simulink model "Series_RLC"  (R2020b)
settings: Solver=VariableStepAuto  StartTime=0.0  StopTime=0.1  RelTol=1e-3
settings Model: Creator=anubh  LastModifiedBy=anubh
settings SFSimCC: CustomCodeUndefinedFunction=UseInterfaceOnly

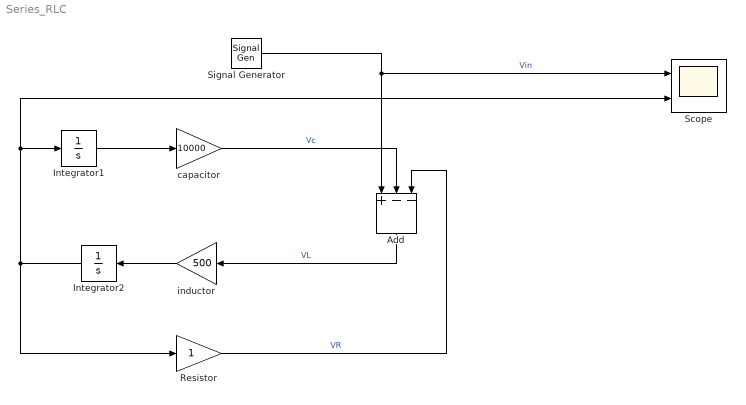
== system Series_RLC ==
  Add : Sum  Inputs=+--
  Integrator1 : Integrator
  Integrator2 : Integrator
  Resistor : Gain
  Scope : Scope  NumInputPorts=2
  Signal Generator : SignalGenerator  WaveForm=square  Amplitude=5  Frequency=1000
  capacitor : Gain  Gain=10000
  inductor : Gain  Gain=500
  wires:
  inductor/1 -> Integrator2/1
  Signal Generator/1 -> Add/1, Scope/1  "Vin"
  Add/1 -> inductor/1  "VL"
  capacitor/1 -> Add/2  "Vc"
  Integrator1/1 -> capacitor/1
  Resistor/1 -> Add/3  "VR"
  Integrator2/1 -> Resistor/1, Scope/2, Integrator1/1
